simulink model "glupi_sistem"  (R2018a)
settings: Solver=VariableStepAuto  StartTime=0.0  StopTime=100  FixedStep=0.001  RelTol=1e-3
settings Model: Creator=Teodor  LastModifiedBy=Teodor

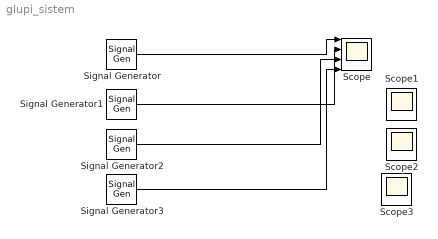
== system glupi_sistem ==
  Scope : Scope  NumInputPorts=4
  Scope1 : Scope
  Scope2 : Scope
  Scope3 : Scope
  Signal Generator : SignalGenerator  Frequency=0.2  Units=rad/sec
  Signal Generator1 : SignalGenerator  WaveForm=square  Frequency=0.2  Units=rad/sec
  Signal Generator2 : SignalGenerator  WaveForm=sawtooth  Frequency=0.2  Units=rad/sec
  Signal Generator3 : SignalGenerator  WaveForm=random  Frequency=0.2  Units=rad/sec
  wires:
  Signal Generator/1 -> Scope/1
  Signal Generator1/1 -> Scope/2
  Signal Generator2/1 -> Scope/3
  Signal Generator3/1 -> Scope/4
